simulink model "test_asbQuadcopter"  (R2021a)
settings: Solver=ode3  StartTime=0  StopTime=10  FixedStep=Ts  RelTol=1e-3  EnableMultiTasking=on
undefined symbols (not defined in the file or in its folder): Command, Desp_XYZ, FinalPos_XYZ, FinalPos_YPR, ft, init, InitPos_XYZ, InitPos_YPR, m, Noise_Amplitude, Noise_Chirp, Noise_Time, Pitch_Noise, Roll_Noise, s, steps_Pitch, steps_Roll, steps_X, steps_Y, steps_Yaw, steps_Z, takeOffDuration, Target_Time, time_stepsX, time_stepsY, time_stepsYaw, time_stepsZ, Time_Trans, Ts, Vehicle, Z_init, Z_Tesp
libraries: simulink x40, aerolibconvert2 x4, aerolibanimutils x2, SignalEditorBlockLib x2, environmentLibrary x2, sensorsLibrary x2, aerolibfltsims x2, aerolibutil x2, vrlib x1
(part 2 of 2)

== system test_asbQuadcopter/Visualization/Visualization/Simulink 3D/Euler to VR/Quaternion Normalization2 ==
  e0 : Inport
  1/2 : Gain  Gain=1/2  SaturateOnIntegerOverflow=on  OutDataTypeStr=Inherit: Same as input  ParamDataTypeStr=Inherit: Same as input
  Demux : Demux  Outputs=[1 3]
      settings: DisplayOption=none
  Mux : Mux  Inputs=2
  Product : Product  InputSameDT=on  SaturateOnIntegerOverflow=on  OutDataTypeStr=Inherit: Same as first input
  Trigonometric Function : Trigonometry
  Trigonometric Function1 : Trigonometry  Operator=cos
  e0_norm : Outport  VectorParamsAs1DForOutWhenUnconnected=off
  wires:
  Trigonometric Function1/1 -> Mux/1
  Demux/2 -> Product/2
  Demux/1 -> 1/2/1
  Mux/1 -> e0_norm/1
  Product/1 -> Mux/2
  Trigonometric Function/1 -> Product/1
  1/2/1 -> Trigonometric Function1/1, Trigonometric Function/1
  e0/1 -> Demux/1

== system test_asbQuadcopter/Command/Signal Editor/Subsystem/Subsystem/Subsystem/Subsystem ==
  Enable : EnablePort
  Band-Limited White Noise : simulink/Sources/Band-Limited White Noise  Cov=[0.01]  Ts=Ts  seed=[23341]
  y : Outport
  wires:
  Band-Limited White Noise/1 -> y/1

== system test_asbQuadcopter/Command/Signal Editor/Subsystem/Subsystem3/Subsystem/Subsystem ==
  Enable : EnablePort
  Band-Limited White Noise : simulink/Sources/Band-Limited White Noise  Cov=[0.01]  Ts=Ts  seed=[23341]
  y : Outport
  wires:
  Band-Limited White Noise/1 -> y/1

== system test_asbQuadcopter/Command/Signal Editor/Subsystem/Subsystem4/Subsystem/Subsystem ==
  Enable : EnablePort
  Band-Limited White Noise : simulink/Sources/Band-Limited White Noise  Cov=[0.01]  Ts=Ts  seed=[23341]
  y : Outport
  wires:
  Band-Limited White Noise/1 -> y/1
